simulink model "KR6_dyn_lib"  (R2018a)
settings: Solver=VariableStepAuto  StartTime=0.0  StopTime=10.0  RelTol=1e-3
(part 1 of 2)
settings Model: Creator=Pedro Ramalho  LastModifiedBy=Pedro Ramalho

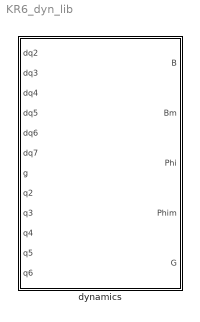
== system KR6_dyn_lib ==
  dynamics : MATLAB Function  TreatAsAtomicUnit=on
